simulink model "KITTRacing"  (R2021a)
settings: Solver=VariableStepAuto  StartTime=0.0  StopTime=10.0  RelTol=1e-3
values from neighbouring files (symbols this model uses):
  b = 0.5    [KITTParameters.m]    (also in controller.m = 5)
  c = 0.01    [KITTParameters.m]    (also in controller.m = 0.1)
  Fa = 0    [KITTDriver.m]    (also in KITTParameters.m = 80; controller.m)
  Fb = 10    [KITTDriver.m]    (also in KITTParameters.m = 0; controller.m = Fbi)
  m = 5.6    [KITTParameters.m]    (also in controller.m)
  s0 = 0    [KITTDriver.m]    (also in KITTParameters.m; controller.m)
  v0 = 10.58    [KITTDriver.m]    (also in KITTParameters.m = 1; controller.m = v0 + (distance - s)*0.6)
settings Model: Creator=flori  LastModifiedBy=flori
settings SolverCC: ZeroCrossAlgorithm=Adaptive
settings DebuggingCC: IgnoredZcDiagnostic=none

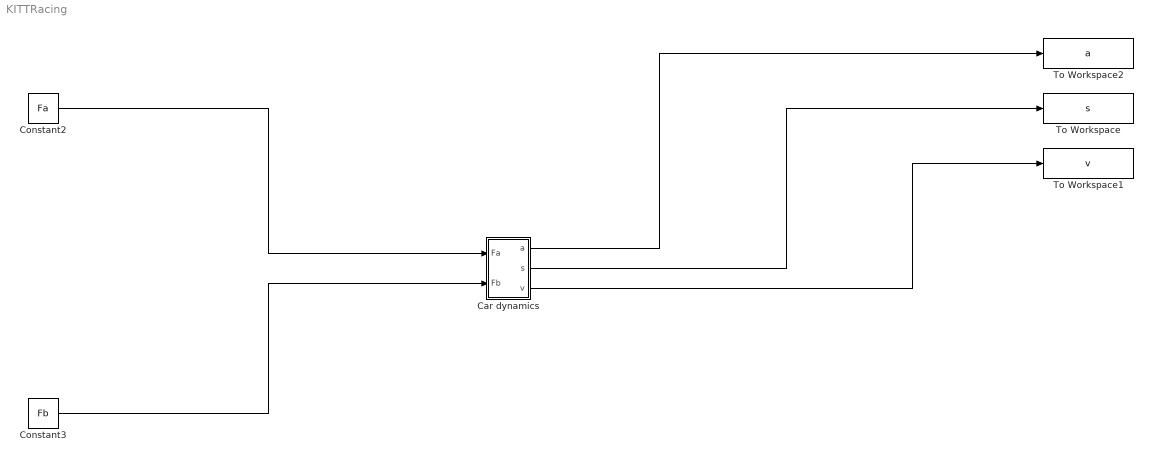
== system KITTRacing ==
  Car dynamics : Subsystem
  Constant2 : Constant  Value=Fa
  Constant3 : Constant  Value=Fb
  To Workspace : ToWorkspace  VariableName=s  SaveFormat=Structure With Time  SampleTime=-1
  To Workspace1 : ToWorkspace  VariableName=v  SaveFormat=Structure With Time  SampleTime=-1
  To Workspace2 : ToWorkspace  VariableName=a  SaveFormat=Structure With Time  SampleTime=-1
  wires:
  Constant2/1 -> Car dynamics/1(Fa)
  Constant3/1 -> Car dynamics/2(Fb)
  Car dynamics/1(a) -> To Workspace2/1
  Car dynamics/2(s) -> To Workspace/1
  Car dynamics/3(v) -> To Workspace1/1

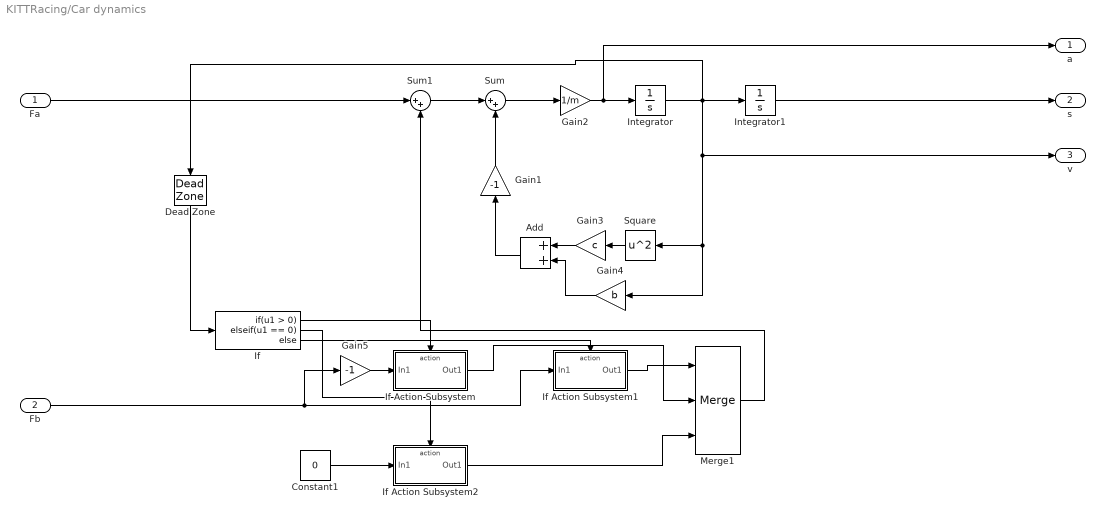
== system KITTRacing/Car dynamics ==
  Fa : Inport
  Fb : Inport  Port=2
  Add : Sum
  Constant1 : Constant  Value=0
  Dead Zone : DeadZone  LowerValue=-0.005  UpperValue=0.005  ZeroCross=off  SaturateOnIntegerOverflow=on
  Gain1 : Gain  Gain=-1
  Gain2 : Gain  Gain=1/m
  Gain3 : Gain  Gain=c
  Gain4 : Gain  Gain=b
  Gain5 : Gain  Gain=-1
  If : If  ElseIfExpressions=u1 == 0
  If Action Subsystem : Subsystem  TreatAsAtomicUnit=on
  If Action Subsystem1 : Subsystem  TreatAsAtomicUnit=on
  If Action Subsystem2 : Subsystem  TreatAsAtomicUnit=on
  Integrator : Integrator  InitialCondition=v0
  Integrator1 : Integrator  InitialCondition=s0
  Merge1 : Merge  Inputs=3
  Square : Math  Operator=square  SaturateOnIntegerOverflow=on
  Sum : Sum  Inputs=|++
  Sum1 : Sum  Inputs=|++
  a : Outport
  s : Outport  Port=2
  v : Outport  Port=3
  wires:
  Add/1 -> Gain1/1
  Fb/1 -> Gain5/1, If Action Subsystem1/1(In1)
  Constant1/1 -> If Action Subsystem2/1(In1)
  Integrator/1 -> Dead Zone/1, v/1, Gain4/1, Square/1, Integrator1/1
  If/2 -> If Action Subsystem2/Action
  If Action Subsystem/1(Out1) -> Merge1/2
  If/1 -> If Action Subsystem/Action
  Gain1/1 -> Sum/2
  Gain2/1 -> a/1, Integrator/1
  Dead Zone/1 -> If/1
  If Action Subsystem2/1(Out1) -> Merge1/3
  Sum/1 -> Gain2/1
  Gain4/1 -> Add/2
  Gain5/1 -> If Action Subsystem/1(In1)
  Sum1/1 -> Sum/1
  If/3 -> If Action Subsystem1/Action
  Gain3/1 -> Add/1
  Square/1 -> Gain3/1
  Merge1/1 -> Sum1/2
  If Action Subsystem1/1(Out1) -> Merge1/1
  Fa/1 -> Sum1/1
  Integrator1/1 -> s/1

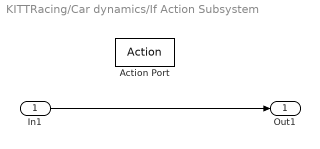
== system KITTRacing/Car dynamics/If Action Subsystem ==
  In1 : Inport
  Action Port : ActionPort  ActionPortLabel=if(u1 > 0)
  Out1 : Outport
  wires:
  In1/1 -> Out1/1

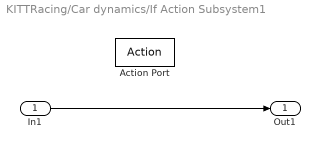
== system KITTRacing/Car dynamics/If Action Subsystem1 ==
  In1 : Inport
  Action Port : ActionPort  ActionPortLabel=else
  Out1 : Outport
  wires:
  In1/1 -> Out1/1

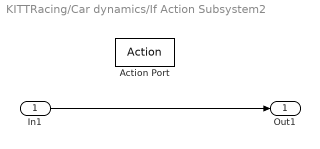
== system KITTRacing/Car dynamics/If Action Subsystem2 ==
  In1 : Inport
  Action Port : ActionPort  ActionPortLabel=elseif(u1 == 0)
  Out1 : Outport
  wires:
  In1/1 -> Out1/1
